simulink library "lib_fuel_cell"  (Simulink 4.00)
undefined symbols (not defined in the file or in its folder): air_cp, amb_tmp, cell_const_F, cell_const_g, cell_const_jo, cell_const_LHV_H2, cell_const_Mair, cell_const_MH, cell_const_MW, cell_const_R2, cell_const_Voc, ex_gas_cp, fan_cool, fc_acc_mass, fc_act, fc_air_comp_map, fc_air_comp_pwr, fc_base_mass, fc_blower_rec_H2, fc_blowera, fc_c2i_th_cond, fc_c_init_tmp, fc_cell_area, fc_cell_const_eta1, fc_cell_const_eta_DCDC, fc_cell_const_etablow, fc_cell_const_etagen, fc_cell_const_etapump, fc_cell_const_ex, fc_cell_const_kw, fc_cell_const_Nrad, fc_cell_const_U, fc_cell_dim_A, fc_cell_dim_tm, fc_cell_num, fc_cell_press_a, fc_cell_press_amb, fc_cell_press_an, fc_cell_press_blowa, fc_cell_press_blowr, fc_cell_press_c, fc_cell_press_hum, fc_cell_press_hyd, fc_cell_stack_dpipe, fc_cell_stack_dpipefc, fc_cell_stack_drad, fc_cell_stack_Lpipe, fc_cell_stack_Lpipefc, fc_cell_stack_Lrad, fc_cell_stack_N, fc_cell_stack_Pel, fc_cell_stoich_RHah, fc_cell_stoich_RHch, fc_cell_stoich_RHo, fc_cell_stoich_vH, fc_cell_stoich_vO, fc_cell_stoich_XON, fc_cell_temp_ah, fc_cell_temp_amb, fc_cell_temp_cell ... (+74)
libraries: fc_vt_lib x2, lib_fuel_cell x1
(part 2 of 5)

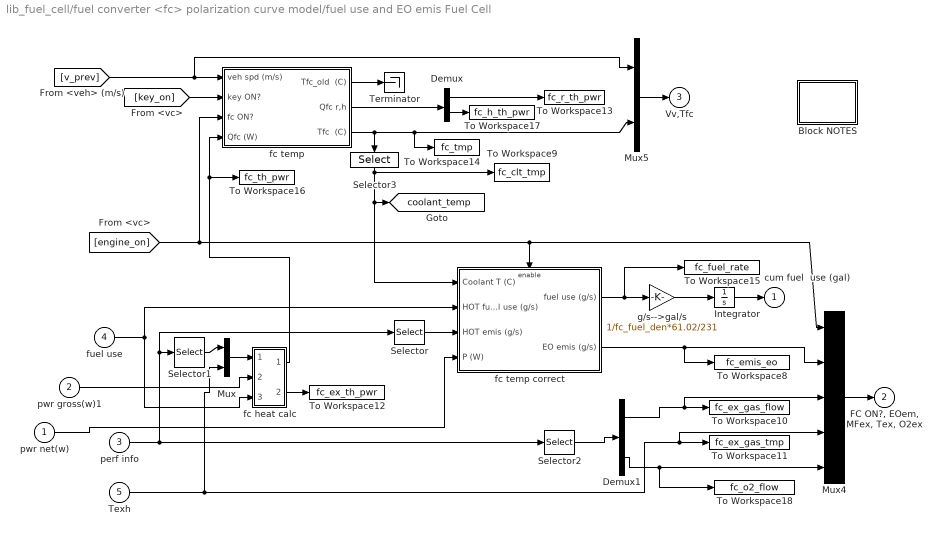
== system lib_fuel_cell/fuel converter <fc> polarization curve model/fuel use and EO emis Fuel Cell ==
  pwr net(w) : Inport  Port=1  LatchInput=off
  pwr gross(w)1 : Inport  Port=2  LatchInput=off
  perf info : Inport  Port=3  LatchInput=off
  fuel use : Inport  Port=4  LatchInput=off
  Texh : Inport  Port=5  LatchInput=off
  Block NOTES : Subsystem
      settings: RTWFcnNameOpts=Auto  RTWFileNameOpts=Auto
      mask Display: disp('Block\nNOTES')
  Demux : Demux  Outputs=2  BusSelectionMode=off
  Demux1 : Demux  Outputs=2  BusSelectionMode=off
  Integrator : Integrator  ExternalReset=none  InitialConditionSource=internal  InitialCondition=0  LimitOutput=off  UpperSaturationLimit=inf  LowerSaturationLimit=-inf  ShowSaturationPort=off  ShowStatePort=off  AbsoluteTolerance=auto
  Mux : Mux  Inputs=2
  Mux4 : Mux  Inputs=[1 4 1 1 1]
      settings: DisplayOption=none
  Mux5 : Mux  Inputs=[1 4 ]
      settings: DisplayOption=none
  Selector : Selector  InputType=Vector  ElementSrc=Internal  Elements=[1 2 3 4]  RowSrc=Internal  Rows=1  ColumnSrc=Internal  Columns=1  InputPortWidth=6
  Selector1 : Selector  InputType=Vector  ElementSrc=Internal  Elements=[5]  RowSrc=Internal  Rows=1  ColumnSrc=Internal  Columns=1  InputPortWidth=6
  Selector2 : Selector  InputType=Vector  ElementSrc=Internal  Elements=[5 6]  RowSrc=Internal  Rows=1  ColumnSrc=Internal  Columns=1  InputPortWidth=6
  Selector3 : Selector  Orientation=down  InputType=Vector  ElementSrc=Internal  Elements=2  RowSrc=Internal  Rows=1  ColumnSrc=Internal  Columns=1  InputPortWidth=4
  Terminator : Terminator
  To Workspace10 : ToWorkspace  VariableName=fc_ex_gas_flow  SampleTime=-1  SaveFormat=Array
  To Workspace11 : ToWorkspace  VariableName=fc_ex_gas_tmp  SampleTime=-1  SaveFormat=Array
  To Workspace12 : ToWorkspace  VariableName=fc_ex_th_pwr  SampleTime=-1  SaveFormat=Array
  To Workspace13 : ToWorkspace  VariableName=fc_r_th_pwr  SampleTime=-1  SaveFormat=Array
  To Workspace14 : ToWorkspace  VariableName=fc_tmp  SampleTime=-1  SaveFormat=Array
  To Workspace15 : ToWorkspace  VariableName=fc_fuel_rate  SampleTime=-1  SaveFormat=Array
  To Workspace16 : ToWorkspace  VariableName=fc_th_pwr  SampleTime=-1  SaveFormat=Array
  To Workspace17 : ToWorkspace  VariableName=fc_h_th_pwr  SampleTime=-1  SaveFormat=Array
  To Workspace18 : ToWorkspace  VariableName=fc_o2_flow  SampleTime=-1  SaveFormat=Array
  To Workspace8 : ToWorkspace  VariableName=fc_emis_eo  SampleTime=-1  SaveFormat=Array
  To Workspace9 : ToWorkspace  VariableName=fc_clt_tmp  SampleTime=-1  SaveFormat=Array
  fc heat calc : Subsystem
      settings: RTWFcnNameOpts=Auto  RTWFileNameOpts=Auto
  fc temp : Subsystem
      settings: RTWFcnNameOpts=Auto  RTWFileNameOpts=Auto
  fc temp correct : Subsystem  TreatAsAtomicUnit=on
      settings: RTWFcnNameOpts=Auto  RTWFileNameOpts=Auto
  g/s-->gal/s : Gain  Gain=1/fc_fuel_den*61.02/231  Multiplication=Element-wise(K.*u)  SaturateOnIntegerOverflow=on
  cum fuel  use (gal) : Outport  Port=1  InitialOutput=0
  "FC ON?, EOem, MFex, Tex, O2ex" : Outport  Port=2  InitialOutput=0
  Vv,Tfc : Outport  Port=3  InitialOutput=0
  tag scope: coolant_temp=global
  wires:
  perf info/1 -> Selector2/1, Selector/1, Selector1/1
  Selector/1 -> fc temp correct/3(HOT emis (g/s))
  fc temp correct/1(fuel use (g/s)) -> To Workspace15/1, g/s-->gal/s/1
  fc temp correct/2(EO emis (g/s)) -> To Workspace8/1, Mux4/2
  g/s-->gal/s/1 -> Integrator/1
  Selector3/1 -> To Workspace9/1, [coolant_temp], fc temp correct/1(Coolant T (C))
  [engine_on] -> fc temp/3(fc ON?), fc temp correct/Enable, Mux4/1
  Integrator/1 -> cum fuel  use (gal)/1
  Mux4/1 -> "FC ON?, EOem, MFex, Tex, O2ex"/1
  fuel use/1 -> fc temp correct/2(HOT fuel use (g/s)), fc heat calc/3(In4)
  [key_on] -> fc temp/2(key ON?)
  Demux/2 -> To Workspace17/1
  Demux/1 -> To Workspace13/1
  fc temp/2(Qfc r,h) -> Demux/1
  fc temp/1(Tfc_old  (C)) -> Terminator/1
  fc temp/3(Tfc  (C)) -> Mux5/2, To Workspace14/1, Selector3/1
  [v_prev] -> fc temp/1(veh spd (m/s)), Mux5/1
  Mux5/1 -> Vv,Tfc/1
  Selector2/1 -> Demux1/1
  Demux1/1 -> To Workspace10/1, Mux4/3
  Texh/1 -> To Workspace11/1, Mux4/4, Mux/2
  Demux1/2 -> To Workspace18/1, Mux4/5
  fc heat calc/2(Out1) -> To Workspace12/1
  fc heat calc/1(Out2) -> fc temp/4(Qfc (W)), To Workspace16/1
  Selector1/1 -> Mux/1
  Mux/1 -> fc heat calc/1(In5)
  pwr net(w)/1 -> fc temp correct/4(P (W))
  pwr gross(w)1/1 -> fc heat calc/2(In3)

== system lib_fuel_cell/fuel converter <fc>  KTH fc model/fuel cell  system <fc>/Block NOTES ==
  note: 7/30/98
      | - started with battery from BD_SER2h.m
      | - added a Saturation block to prevent computed
      |        SOC from falling below 0 or rising above 1
      | - added logic in 'limit power' to prevent discharge
      | if SOC is below 0.001 (0.1%)
      | -added limit block to check if low SOC is preventing
      | discharge
  note: Power loss is computed as I*R+losses due to Coulombic (in)efficiency.
  note: This block models the energy storage system as an SOC-dependent voltage
      | in series with an SOC- and current direction-dependent internal resistance.
      | SOC is computed assuming that A-h capacity is a function of average discharge
      | current:  (A-h capacity)=ess_peukert_coeff * (average discharge current)^ess_peukert_exp.
      |
      | Discharge power is limited here so as not to bring the bus (battery pack) voltage below
      | the minimum controller voltage and so as to allow the solution of the quadratic eq'n for
      | discharge current.
      |
      | Positive current is discharge current in the convention used here.

== system lib_fuel_cell/fuel converter <fc>  KTH fc model/fuel cell  system <fc>/KTH fc model ==
  note: KTH Fuel Cell System
      | (PEM Fuel Cell)
  note: W/ re-circulation of hydrogen
  In1 : Inport  Port=1  LatchInput=off
  Enable : EnablePort  StatesWhenEnabling=reset
  Fcn : Fcn  Expr=u(6)
  PEM fuel cell system : Subsystem
      settings: RTWFcnNameOpts=Auto  RTWFileNameOpts=Auto
  emissions info : Subsystem
      settings: RTWFcnNameOpts=Auto  RTWFileNameOpts=Auto
  pwr avail. to driveline (W) : Outport  Port=1  InitialOutput=0
  Emissions info : Outport  Port=2
  fuel use : Outport  Port=3  InitialOutput=0
  system characteristics : Outport  Port=4
  wires:
  In1/1 -> PEM fuel cell system/1("Power request from drivetrain [W] ")
  emissions info/1(emission info CO HC NOx PM mass flow exhaust exhaust temperature O2) -> Emissions info/1
  PEM fuel cell system/1(Pnet [W]) -> pwr avail. to driveline (W)/1
  PEM fuel cell system/2(System characteristics) -> Fcn/1, system characteristics/1
  Fcn/1 -> fuel use/1

== system lib_fuel_cell/fuel converter <fc>  KTH fc model/fuel use and EO emis Fuel Cell/Block NOTES ==
  note: This block determines actual fuel use and engine-out emissions
      | given the fully hot values and the engine coolant temperature.
      | The correlations used here were developed at NREL using
      | FTP data collected under subcontract by JDM & Associates.
      | Note: PM hot/cold relation assumed same as HC

== system lib_fuel_cell/fuel converter <fc> GCTool linkage/fuel cell  system <fc>/Block NOTES ==
  note: 7/30/98
      | - started with battery from BD_SER2h.m
      | - added a Saturation block to prevent computed
      |        SOC from falling below 0 or rising above 1
      | - added logic in 'limit power' to prevent discharge
      | if SOC is below 0.001 (0.1%)
      | -added limit block to check if low SOC is preventing
      | discharge
  note: Power loss is computed as I*R+losses due to Coulombic (in)efficiency.
  note: This block models the energy storage system as an SOC-dependent voltage
      | in series with an SOC- and current direction-dependent internal resistance.
      | SOC is computed assuming that A-h capacity is a function of average discharge
      | current:  (A-h capacity)=ess_peukert_coeff * (average discharge current)^ess_peukert_exp.
      |
      | Discharge power is limited here so as not to bring the bus (battery pack) voltage below
      | the minimum controller voltage and so as to allow the solution of the quadratic eq'n for
      | discharge current.
      |
      | Positive current is discharge current in the convention used here.

== system lib_fuel_cell/fuel converter <fc> GCTool linkage/fuel cell  system <fc>/GCTool fuel cell model ==
  note: Demux Port Labels:
      | net pwr (W)
      | hc (g/s)
      | co (g/s)
      | nox (g/s)
      | pm (g/s)
      | MFexh (g/s)
      | Texh (C)
      | O2 (g/s), dummy
      | ???
      | ???
      | ???
      | fuel use (kg/s)
  net pwr req (W) : Inport  Port=1  LatchInput=off
  Enable : EnablePort  StatesWhenEnabling=reset
  Demux : Demux  Outputs=11  BusSelectionMode=off
  GCTool  Fuel Cell Model : Subsystem  mask(GCTool Fuel Cell Model){x=1, y=2, z=3}
      mask prompts: x "param1:"; y "param2:"; z "param3:"
      mask help: This block will call the GCTool fuel cell modeling software to determine the output parameters of the fuel cell.
      settings: RTWFcnNameOpts=Auto  RTWFileNameOpts=Auto
  Ground : Ground
  Memory : Memory  Orientation=left  X0=[0 0 0]  InheritSampleTime=off
      settings: RTWStateStorageClass=Auto
  Mux5 : Mux  Inputs=7
      settings: DisplayOption=none
  Mux6 : Mux  Inputs=2
      settings: DisplayOption=none
  Mux7 : Mux  Inputs=3
      settings: DisplayOption=none
  net pwr out (W) : Outport  Port=1  OutputWhenDisabled=reset  InitialOutput=0
  emis info hc co nox pm MFexh Texh O2 : Outport  Port=2
  fuel use : Outport  Port=3  OutputWhenDisabled=reset  InitialOutput=0
  wires:
  Ground/1 -> Mux5/7
  Demux/11 -> fuel use/1
  Mux7/1 -> Memory/1
  Demux/10 -> Mux7/3
  Demux/9 -> Mux7/2
  Demux/8 -> Mux7/1
  Demux/7 -> Mux5/6
  Mux5/1 -> emis info hc co nox pm MFexh Texh O2/1
  Demux/6 -> Mux5/5
  Demux/5 -> Mux5/4
  Demux/4 -> Mux5/3
  Demux/3 -> Mux5/2
  Demux/2 -> Mux5/1
  Demux/1 -> net pwr out (W)/1
  Memory/1 -> Mux6/2
  Mux6/1 -> GCTool  Fuel Cell Model/1(In1)
  net pwr req (W)/1 -> Mux6/1
  GCTool  Fuel Cell Model/1(Out1) -> Demux/1

== system lib_fuel_cell/fuel converter <fc> GCTool linkage/fuel use and EO emis Fuel Cell/Block NOTES ==
  note: This block determines actual fuel use and engine-out emissions
      | given the fully hot values and the engine coolant temperature.
      | The correlations used here were developed at NREL using
      | FTP data collected under subcontract by JDM & Associates.
      | Note: PM hot/cold relation assumed same as HC

== system lib_fuel_cell/fuel converter <fc> GCTool linkage/fuel use and EO emis Fuel Cell/fc heat calc ==
  In5 : Inport  Port=1  LatchInput=off
  In3 : Inport  Port=2  LatchInput=off
  In4 : Inport  Port=3  LatchInput=off
  Fcn3 : Fcn  Expr=(u(1)/1000)*ex_gas_cp*(u(2) - amb_tmp)
  MinMax : MinMax  Function=min  Inputs=2
  Sum5 : Sum  Inputs=-+  SaturateOnIntegerOverflow=on
  Sum6 : Sum  Inputs=-+  SaturateOnIntegerOverflow=on
  lhv : Gain  Gain=fc_fuel_lhv  Multiplication=Element-wise(K.*u)  SaturateOnIntegerOverflow=on
  Out2 : Outport  Port=1  InitialOutput=0
  Out1 : Outport  Port=2  InitialOutput=0
  wires:
  In5/1 -> Fcn3/1
  Fcn3/1 -> MinMax/1
  Sum6/1 -> Sum5/2, MinMax/2
  lhv/1 -> Sum6/2
  Sum5/1 -> Out2/1
  In3/1 -> Sum6/1
  In4/1 -> lhv/1
  MinMax/1 -> Sum5/1, Out1/1

== system lib_fuel_cell/fuel converter <fc> GCTool linkage/fuel use and EO emis Fuel Cell/fc temp ==
  note: c
  note: i
  note: x
  note: h
  veh spd (m/s) : Inport  Port=1  LatchInput=off
  key ON? : Inport  Orientation=down  Port=2  LatchInput=off
  fc ON? : Inport  Port=3  LatchInput=off
  Qfc (W) : Inport  Port=4  LatchInput=off
  1/ : Gain  Gain=1/(0.2*fc_base_mass*fc_pwr_scale*fc_cp)  Multiplication=Element-wise(K.*u)  SaturateOnIntegerOverflow=on
  1/Ci : Gain  Gain=1/(0.8*fc_base_mass*fc_pwr_scale*fc_cp)  Multiplication=Element-wise(K.*u)  SaturateOnIntegerOverflow=on
  1/Cx : Gain  Gain=1/(fc_acc_mass*fc_pwr_scale*fc_cp)  Multiplication=Element-wise(K.*u)  SaturateOnIntegerOverflow=on
  1/mcp : Gain  Gain=1/(0.1*veh_glider_mass*fc_pwr_scale*fc_h_cp)  Multiplication=Element-wise(K.*u)  SaturateOnIntegerOverflow=on
  Block NOTES : Subsystem
      settings: RTWFcnNameOpts=Auto  RTWFileNameOpts=Auto
      mask Display: disp('Block\nNOTES')
  Mux3 : Mux  Inputs=4
      settings: DisplayOption=none
  Mux4 : Mux  Inputs=2
      settings: DisplayOption=none
  Qc : Sum  Inputs=++  SaturateOnIntegerOverflow=on
  Qc1 : Sum  Inputs=--+  SaturateOnIntegerOverflow=on
  Tcm : Integrator  ExternalReset=none  InitialConditionSource=internal  InitialCondition=fc_c_init_tmp  LimitOutput=off  UpperSaturationLimit=inf  LowerSaturationLimit=-inf  ShowSaturationPort=off  ShowStatePort=off  AbsoluteTolerance=auto
  Tcx : Integrator  ExternalReset=none  InitialConditionSource=internal  InitialCondition=fc_x_init_tmp  LimitOutput=off  UpperSaturationLimit=inf  LowerSaturationLimit=-inf  ShowSaturationPort=off  ShowStatePort=off  AbsoluteTolerance=auto
  Tcx1 : Integrator  ExternalReset=none  InitialConditionSource=internal  InitialCondition=fc_i_init_tmp  LimitOutput=off  UpperSaturationLimit=inf  LowerSaturationLimit=-inf  ShowSaturationPort=off  ShowStatePort=off  AbsoluteTolerance=auto
  Tm : Integrator  ExternalReset=none  InitialConditionSource=internal  InitialCondition=fc_h_init_tmp  LimitOutput=off  UpperSaturationLimit=inf  LowerSaturationLimit=-inf  ShowSaturationPort=off  ShowStatePort=off  AbsoluteTolerance=auto
  fc coolant : Subsystem  TreatAsAtomicUnit=on
      settings: RTWFcnNameOpts=Auto  RTWFileNameOpts=Auto
  fc mass heat flow : Subsystem
      settings: RTWFcnNameOpts=Auto  RTWFileNameOpts=Auto
  old fc coolant  temp. (C) : Subsystem
      settings: RTWFcnNameOpts=Auto  RTWFileNameOpts=Auto
  Tfc_old  (C) : Outport  Port=1  InitialOutput=0
  Qfc r,h : Outport  Port=2  InitialOutput=0
  Tfc  (C) : Outport  Port=3  InitialOutput=0
  wires:
  fc ON?/1 -> old fc coolant  temp. (C)/1(fc on?)
  veh spd (m/s)/1 -> fc mass heat flow/1(veh spd), old fc coolant  temp. (C)/2(veh spd)
  old fc coolant  temp. (C)/1(fc coolant  temp (C)) -> Tfc_old  (C)/1
  Mux3/1 -> Tfc  (C)/1, fc mass heat flow/2(fc_temp)
  fc mass heat flow/4(Qfc_h) -> 1/mcp/1
  1/mcp/1 -> Tm/1
  Tm/1 -> Mux3/4
  Tcx/1 -> Mux3/3
  key ON?/1 -> fc coolant/Enable
  fc mass heat flow/3(Qfc_x) -> 1/Cx/1
  1/Cx/1 -> Tcx/1
  Mux4/1 -> Qfc r,h/1
  Tcx1/1 -> Mux3/2, fc coolant/1(Tcl)
  fc coolant/1(Qfc_rad) -> Mux4/1, Qc1/1
  fc coolant/2(Qfc_htr) -> Mux4/2, Qc1/2
  fc mass heat flow/2(Qfc_i) -> fc coolant/2("Qfc_i "), Qc1/3
  Tcm/1 -> Mux3/1
  1/Ci/1 -> Tcx1/1
  Qc1/1 -> 1/Ci/1
  fc mass heat flow/1(Qfc_c) -> Qc/2
  Qfc (W)/1 -> Qc/1
  1//1 -> Tcm/1
  Qc/1 -> 1//1

== system lib_fuel_cell/fuel converter <fc> VT model/Fuel Cell Power System Model (S. Gurski - Virgina Tech)/Algebraic Constraint1 ==
  f(z) : Inport  Port=1  LatchInput=off
  Initial Guess : InitialCondition  Value=z0
  Sum : Sum  Inputs=|++  SaturateOnIntegerOverflow=on
  z : Outport  Port=1
  wires:
  Sum/1 -> Initial Guess/1
  Initial Guess/1 -> Sum/2, z/1
  f(z)/1 -> Sum/1

== system lib_fuel_cell/fuel converter <fc> VT model/Fuel Cell Power System Model (S. Gurski - Virgina Tech)/Bus Creator ==
  In1 : Inport  Port=1  LatchInput=off
  Bus Creator : BusCreator  Inputs=59
  Demux : Demux  Outputs=59  BusSelectionMode=off
  system_characteristics : Outport  Port=1
  wires:
  Demux/30 -> Bus Creator/30  "water_balance"
  Demux/29 -> Bus Creator/29  "condenser_working_capacity"
  Demux/28 -> Bus Creator/28  "cell_voltage"
  Demux/23 -> Bus Creator/23  "mwv_anode_inlet"
  Demux/24 -> Bus Creator/24  "mwv_cathode_inlet"
  Demux/25 -> Bus Creator/25  "water_gen"
  Demux/26 -> Bus Creator/26  "mwv_cathode_outlet"
  Demux/27 -> Bus Creator/27  "condenser_recovered_water"
  Demux/1 -> Bus Creator/1  "fc_gross_power_gen"
  Demux/2 -> Bus Creator/2  "air_compressor_power"
  Demux/3 -> Bus Creator/3  "condenser_fan_power"
  Demux/4 -> Bus Creator/4  "radiator_fan_power"
  Demux/5 -> Bus Creator/5  "coolant_pump_power"
  Demux/6 -> Bus Creator/6  "m_dot_air"
  Demux/7 -> Bus Creator/7  "m_dot_coolant"
  Demux/8 -> Bus Creator/8  "pressure_inlet_cathode"
  Demux/9 -> Bus Creator/9  "fc_cell_current"
  Demux/10 -> Bus Creator/10  "m_dot_h2"
  Demux/11 -> Bus Creator/11  "q_gen_stack"
  Demux/12 -> Bus Creator/12  "t_stack_coolant_in"
  Demux/13 -> Bus Creator/13  "t_stack_coolant_output"
  Demux/14 -> Bus Creator/14  "t_humidifier_coolant_out"
  Demux/15 -> Bus Creator/15  "t_radiator_coolant_out"
  Demux/16 -> Bus Creator/16  "condenser_heat_to_ambient"
  Demux/17 -> Bus Creator/17  "radiator_energy_loss_ambient"
  Demux/18 -> Bus Creator/18  "stack_energy_loss_ambient"
  Demux/19 -> Bus Creator/19  "reservoir_energy_loss_ambient"
  Demux/20 -> Bus Creator/20  "air_compressor_speed"
  Demux/21 -> Bus Creator/21  "air_compressor_adiabatic_efficiency"
  Demux/22 -> Bus Creator/22  "air_compressor_volumetric_efficiency"
  In1/1 -> Demux/1
  Bus Creator/1 -> system_characteristics/1
  Demux/31 -> Bus Creator/31  "condensed_water_in_stack"
  Demux/32 -> Bus Creator/32  "m_dot_h2o_anode"
  Demux/33 -> Bus Creator/33  "m_dot_h2o_cathode"
  Demux/34 -> Bus Creator/34  "stack_heat_loads1"
  Demux/35 -> Bus Creator/35  "stack_heat_loads2"
  Demux/36 -> Bus Creator/36  "stack_heat_loads3"
  Demux/37 -> Bus Creator/37  "stack_heat_loads4"
  Demux/38 -> Bus Creator/38  "stack_heat_loads5"
  Demux/39 -> Bus Creator/39  "stack_heat_loads6"
  Demux/40 -> Bus Creator/40  "stack_heat_loads7"
  Demux/41 -> Bus Creator/41  "stack_heat_loads8"
  Demux/42 -> Bus Creator/42  "stack_heat_loads9"
  Demux/43 -> Bus Creator/43  "Q_humidifier"
  Demux/44 -> Bus Creator/44  "cell_efficiency"
  Demux/45 -> Bus Creator/45  "system_efficiency"
  Demux/46 -> Bus Creator/46  "exhaust_m_dot_water"
  Demux/47 -> Bus Creator/47  "exhaust_heat_loss"
  Demux/48 -> Bus Creator/48  "exhaust_quality"
  Demux/49 -> Bus Creator/49  "oxygen_partial_pressure"
  Demux/50 -> Bus Creator/50  "pressure_ratio"
  Demux/51 -> Bus Creator/51  "operating_pressure"
  Demux/52 -> Bus Creator/52  "m_dot_air_out"
  Demux/53 -> Bus Creator/53  "by_pass_energy_loss_ambient"
  Demux/54 -> Bus Creator/54  "o2_pp_inlet"
  Demux/55 -> Bus Creator/55  "o2_pp_outlet"
  Demux/56 -> Bus Creator/56  "psat"
  Demux/57 -> Bus Creator/57  "t_compresser_out"
  Demux/58 -> Bus Creator/58  "t_reservoir_coolant_out"
  Demux/59 -> Bus Creator/59  "o2_percent"

== system lib_fuel_cell/fuel converter <fc> VT model/Fuel Cell Power System Model (S. Gurski - Virgina Tech)/Fuel Cell System ==
  In1 : Inport  Port=1  LatchInput=off
  Action Port : ActionPort  InitializeStates=held  ActionType=unset
  Algebraic Constraint : Subsystem  AncestorBlock=simulink3/Math/Algebraic Constraint  mask(Algebraic Constraint){z0=0.3}
      mask prompts: z0 "Initial guess:"
      mask help: Constrains input signal f(z) to zero and outputs an algebraic state z. This block outputs the value necessary to produce a zero at the input. The output must affect the input through some feedback path. Provide an initial guess of the output to improve algebraic loop solver efficiency.
      settings: RTWFcnNameOpts=Auto  RTWFileNameOpts=Auto
      mask Help:
      | This block outputs the value necessary to produce a zero at the input. The output must affect the input through some feedback path. This allows you to specify algebraic equations for index 1 differential/algebraic systems (DAE's).
      | 
      | By default, the initial guess is zero.  You can improve the efficiency of the algebraic loop solver by providing an initial guess that is close to the solution value.
      mask Display: disp('Solve\nf(z) = 0')
  Constant : Constant  Value=1
  Demux1 : Demux  Outputs=6  BusSelectionMode=off
  Fuel Cell System : Subsystem
      settings: RTWFcnNameOpts=Auto  RTWFileNameOpts=Auto
  Mux : Mux  Inputs=6
  Sum : Sum  Inputs=|+-  SaturateOnIntegerOverflow=on
  Out1 : Outport  Port=1  OutputWhenDisabled=reset  InitialOutput=0
  Out2 : Outport  Port=2  OutputWhenDisabled=reset  InitialOutput=0
  wires:
  Algebraic Constraint/1(z) -> Fuel Cell System/1(" Current Density Request")
  Sum/1 -> Algebraic Constraint/1(f(z))
  Mux/1 -> Out1/1
  In1/1 -> Demux1/1
  Demux1/1 -> Sum/1
  Demux1/2 -> Fuel Cell System/2(t_stack_coolant_in1)
  Demux1/3 -> Fuel Cell System/3(fc_stack_temperature)
  Demux1/4 -> Fuel Cell System/4(water_balance_previous)
  Fuel Cell System/1(Net Power Gen) -> Mux/1, Sum/2
  Fuel Cell System/2(Stack Temperature) -> Mux/2
  Fuel Cell System/3(cell_voltage) -> Mux/3
  Fuel Cell System/4(t_stack_coolant_in) -> Mux/4
  Fuel Cell System/5(waterbalance) -> Mux/5
  Constant/1 -> Out2/1
  Fuel Cell System/6(system_characteristics) -> Mux/6
  Demux1/5 -> Fuel Cell System/5(elevation)
  Demux1/6 -> Fuel Cell System/6(vehicle speed (m/s))

== system lib_fuel_cell/fuel converter <fc> VT model/Fuel Cell Power System Model (S. Gurski - Virgina Tech)/Fuel Cell System - min voltage ==
  " Current Density Request" : Inport  Port=1  LatchInput=off
  t_stack_coolant_in1 : Inport  Port=2  LatchInput=off
  fc_stack_temperature : Inport  Port=3  LatchInput=off
  water_balance_previous : Inport  Port=4  LatchInput=off
  elevation : Inport  Port=5  LatchInput=off
  vehicle speed (m/s) : Inport  Port=6  LatchInput=off
  Main Loop - min voltage : fc_vt_lib/Main Loop - min voltage
      settings: RTWFcnNameOpts=Auto  RTWFileNameOpts=Auto
  Net Power Gen : Outport  Port=1
  Stack Temperature : Outport  Port=2
  cell_voltage : Outport  Port=3
  t_stack_coolant_in : Outport  Port=4
  waterbalance : Outport  Port=5
  system_characteristics : Outport  Port=6
  wires:
  elevation/1 -> Main Loop - min voltage/5
  Main Loop - min voltage/6 -> system_characteristics/1
  water_balance_previous/1 -> Main Loop - min voltage/4
  fc_stack_temperature/1 -> Main Loop - min voltage/3
  t_stack_coolant_in1/1 -> Main Loop - min voltage/2
  Main Loop - min voltage/5 -> cell_voltage/1
  " Current Density Request"/1 -> Main Loop - min voltage/1
  Main Loop - min voltage/2 -> waterbalance/1
  Main Loop - min voltage/3 -> Stack Temperature/1
  Main Loop - min voltage/4 -> t_stack_coolant_in/1
  Main Loop - min voltage/1 -> Net Power Gen/1
  vehicle speed (m/s)/1 -> Main Loop - min voltage/6

== system lib_fuel_cell/fuel converter <fc> VT model/fuel use and EO emis Fuel Cell/Block NOTES ==
  note: This block determines actual fuel use and engine-out emissions
      | given the fully hot values and the engine coolant temperature.
      | The correlations used here were developed at NREL using
      | FTP data collected under subcontract by JDM & Associates.
      | Note: PM hot/cold relation assumed same as HC

== system lib_fuel_cell/fuel converter <fc> net model/fuel cell  system <fc>/Block NOTES ==
  note: 7/30/98
      | - started with battery from BD_SER2h.m
      | - added a Saturation block to prevent computed
      |        SOC from falling below 0 or rising above 1
      | - added logic in 'limit power' to prevent discharge
      | if SOC is below 0.001 (0.1%)
      | -added limit block to check if low SOC is preventing
      | discharge
  note: Power loss is computed as I*R+losses due to Coulombic (in)efficiency.
  note: This block models the energy storage system as an SOC-dependent voltage
      | in series with an SOC- and current direction-dependent internal resistance.
      | SOC is computed assuming that A-h capacity is a function of average discharge
      | current:  (A-h capacity)=ess_peukert_coeff * (average discharge current)^ess_peukert_exp.
      |
      | Discharge power is limited here so as not to bring the bus (battery pack) voltage below
      | the minimum controller voltage and so as to allow the solution of the quadratic eq'n for
      | discharge current.
      |
      | Positive current is discharge current in the convention used here.

== system lib_fuel_cell/fuel converter <fc> net model/fuel cell  system <fc>/pwr vs. eff  fuel cell model ==
  net pwr req (W) : Inport  Port=1  LatchInput=off
  Enable : EnablePort  StatesWhenEnabling=reset
  enforce limits : Subsystem
      settings: RTWFcnNameOpts=Auto  RTWFileNameOpts=Auto
  net pwr avail (W) : Outport  Port=1  OutputWhenDisabled=reset  InitialOutput=0
  wires:
  enforce limits/1(Out1) -> net pwr avail (W)/1
  net pwr req (W)/1 -> enforce limits/1(In1)

== system lib_fuel_cell/fuel converter <fc> net model/fuel use and EO emis Fuel Cell/Block NOTES ==
  note: This block determines actual fuel use and engine-out emissions
      | given the fully hot values and the engine coolant temperature.
      | The correlations used here were developed at NREL using
      | FTP data collected under subcontract by JDM & Associates.
      | Note: PM hot/cold relation assumed same as HC

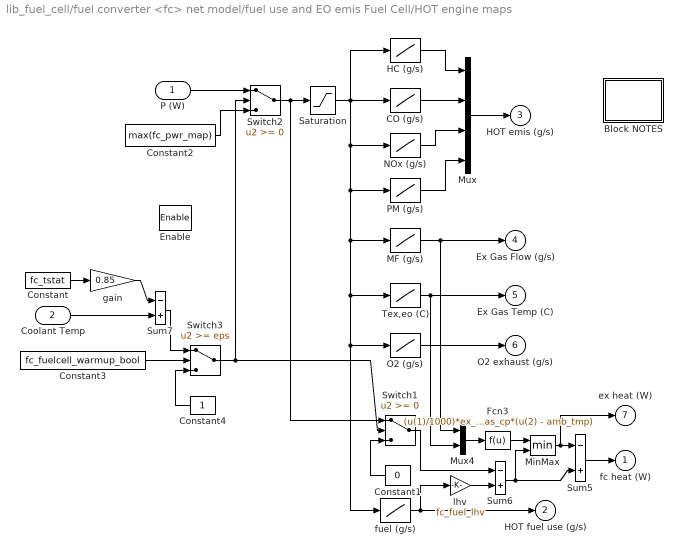
== system lib_fuel_cell/fuel converter <fc> net model/fuel use and EO emis Fuel Cell/HOT engine maps  ==
  P (W) : Inport  Port=1  LatchInput=off
  Coolant Temp : Inport  Port=2  LatchInput=off
  Enable : EnablePort  StatesWhenEnabling=reset
  Block NOTES : Subsystem
      settings: RTWFcnNameOpts=Auto  RTWFileNameOpts=Auto
      mask Display: disp('Block\nNOTES')
  CO (g/s) : Lookup  InputValues=fc_pwr_map*fc_pwr_scale  OutputValues=fc_co_map*fc_pwr_scale
  Constant : Constant  Value=fc_tstat
  Constant1 : Constant  Orientation=left  Value=0
  Constant2 : Constant  Value=max(fc_pwr_map)
  Constant3 : Constant  Value=fc_fuelcell_warmup_bool
  Constant4 : Constant  Orientation=left  Value=1
  Fcn3 : Fcn  Expr=(u(1)/1000)*ex_gas_cp*(u(2) - amb_tmp)
  HC (g/s) : Lookup  InputValues=fc_pwr_map*fc_pwr_scale  OutputValues=fc_hc_map*fc_pwr_scale
  MF (g/s) : Lookup  InputValues=fc_pwr_map*fc_pwr_scale  OutputValues=fc_exflow_map*fc_pwr_scale
  MinMax : MinMax  Function=min  Inputs=2
  Mux : Mux  Inputs=4
      settings: DisplayOption=none
  Mux4 : Mux  Inputs=2
      settings: DisplayOption=none
  NOx (g/s) : Lookup  InputValues=fc_pwr_map*fc_pwr_scale  OutputValues=fc_nox_map*fc_pwr_scale
  O2 (g/s) : Lookup  InputValues=fc_pwr_map*fc_pwr_scale  OutputValues=fc_o2_map*fc_pwr_scale
  PM (g/s) : Lookup  InputValues=fc_pwr_map*fc_pwr_scale  OutputValues=fc_pm_map*fc_pwr_scale
  Saturation : Saturate  UpperLimit=max(fc_pwr_map*fc_pwr_scale)  LowerLimit=0  LinearizeAsGain=on
  Sum5 : Sum  Inputs=-+  SaturateOnIntegerOverflow=on
  Sum6 : Sum  Inputs=-+  SaturateOnIntegerOverflow=on
  Sum7 : Sum  Inputs=-+  SaturateOnIntegerOverflow=on
  Switch1 : Switch  Threshold=0
  Switch2 : Switch  Threshold=0
  Switch3 : Switch  Threshold=eps
  Tex,eo (C) : Lookup  InputValues=fc_pwr_map*fc_pwr_scale  OutputValues=fc_extmp_map
  fuel (g/s) : Lookup  InputValues=fc_pwr_map*fc_pwr_scale  OutputValues=fc_fuel_map*fc_pwr_scale/fc_eff_scale
  gain : Gain  Gain=0.85  Multiplication=Element-wise(K.*u)  SaturateOnIntegerOverflow=on
  lhv : Gain  Gain=fc_fuel_lhv  Multiplication=Element-wise(K.*u)  SaturateOnIntegerOverflow=on
  fc heat (W) : Outport  Port=1  OutputWhenDisabled=reset  InitialOutput=eps
  HOT fuel use (g/s) : Outport  Port=2  OutputWhenDisabled=reset  InitialOutput=eps
  HOT emis (g/s) : Outport  Port=3  OutputWhenDisabled=reset  InitialOutput=eps
  Ex Gas Flow (g/s) : Outport  Port=4  OutputWhenDisabled=reset  InitialOutput=eps
  Ex Gas Temp (C) : Outport  Port=5  OutputWhenDisabled=reset  InitialOutput=amb_tmp
  O2 exhaust (g/s) : Outport  Port=6  OutputWhenDisabled=reset  InitialOutput=eps
  ex heat (W) : Outport  Port=7  OutputWhenDisabled=reset  InitialOutput=eps
  wires:
  O2 (g/s)/1 -> O2 exhaust (g/s)/1
  fuel (g/s)/1 -> lhv/1, HOT fuel use (g/s)/1
  Constant1/1 -> Switch1/3
  lhv/1 -> Sum6/2
  Sum6/1 -> MinMax/2, Sum5/2
  MinMax/1 -> ex heat (W)/1, Sum5/1
  Fcn3/1 -> MinMax/1
  Sum5/1 -> fc heat (W)/1
  Mux4/1 -> Fcn3/1
  Switch1/1 -> Sum6/1
  CO (g/s)/1 -> Mux/2
  Saturation/1 -> HC (g/s)/1, NOx (g/s)/1, PM (g/s)/1, O2 (g/s)/1, fuel (g/s)/1, Tex,eo (C)/1, MF (g/s)/1, CO (g/s)/1
  Tex,eo (C)/1 -> Mux4/2, Ex Gas Temp (C)/1
  MF (g/s)/1 -> Mux4/1, Ex Gas Flow (g/s)/1
  Mux/1 -> HOT emis (g/s)/1
  NOx (g/s)/1 -> Mux/3
  HC (g/s)/1 -> Mux/1
  PM (g/s)/1 -> Mux/4
  P (W)/1 -> Switch2/1
  Constant2/1 -> Switch2/3
  Switch2/1 -> Saturation/1, Switch1/1
  Switch3/1 -> Switch1/2, Switch2/2
  Constant3/1 -> Switch3/2
  Sum7/1 -> Switch3/1
  gain/1 -> Sum7/1
  Coolant Temp/1 -> Sum7/2
  Constant/1 -> gain/1
  Constant4/1 -> Switch3/3

== system lib_fuel_cell/fuel converter <fc> net model/fuel use and EO emis Fuel Cell/System  Efficiency ==
  In1 : Inport  Port=1  LatchInput=off
  Constant : Constant  Value=eps
  Gain : Gain  Gain=fc_fuel_lhv  Multiplication=Element-wise(K.*u)  SaturateOnIntegerOverflow=on
  Gain1 : Gain  Gain=100  Multiplication=Element-wise(K.*u)  SaturateOnIntegerOverflow=on
  Product : Product  Inputs=*/  Multiplication=Element-wise(.*)  SaturateOnIntegerOverflow=on
  Sum1 : Sum  Inputs=|++  SaturateOnIntegerOverflow=on
  To Workspace1 : ToWorkspace  VariableName=fc_eff_out_a  SampleTime=-1  SaveFormat=Array
  tag scope: fc_eff_out_a=global
  wires:
  [fc_pwr_out_a] -> Product/1
  Product/1 -> Gain1/1
  Gain/1 -> Sum1/1
  Constant/1 -> Sum1/2
  Sum1/1 -> Product/2
  Gain1/1 -> To Workspace1/1, [fc_eff_out_a]
  In1/1 -> Gain/1

== system lib_fuel_cell/fuel converter <fc> net model/fuel use and EO emis Fuel Cell/fc temp ==
  note: c
  note: i
  note: x
  note: h
  veh spd (m/s) : Inport  Port=1  LatchInput=off
  key ON? : Inport  Orientation=down  Port=2  LatchInput=off
  fc ON? : Inport  Port=3  LatchInput=off
  Qfc (W) : Inport  Port=4  LatchInput=off
  1/ : Gain  Gain=1/(0.2*fc_base_mass*fc_pwr_scale*fc_cp)  Multiplication=Element-wise(K.*u)  SaturateOnIntegerOverflow=on
  1/Ci : Gain  Gain=1/(0.8*fc_base_mass*fc_pwr_scale*fc_cp)  Multiplication=Element-wise(K.*u)  SaturateOnIntegerOverflow=on
  1/Cx : Gain  Gain=1/(fc_acc_mass*fc_pwr_scale*fc_cp)  Multiplication=Element-wise(K.*u)  SaturateOnIntegerOverflow=on
  1/mcp : Gain  Gain=1/(0.1*veh_glider_mass*fc_pwr_scale*fc_h_cp)  Multiplication=Element-wise(K.*u)  SaturateOnIntegerOverflow=on
  Block NOTES : Subsystem
      settings: RTWFcnNameOpts=Auto  RTWFileNameOpts=Auto
      mask Display: disp('Block\nNOTES')
  Mux3 : Mux  Inputs=4
      settings: DisplayOption=none
  Mux4 : Mux  Inputs=2
      settings: DisplayOption=none
  Qc : Sum  Inputs=++  SaturateOnIntegerOverflow=on
  Qc1 : Sum  Inputs=--+  SaturateOnIntegerOverflow=on
  Tcm : Integrator  ExternalReset=none  InitialConditionSource=internal  InitialCondition=fc_c_init_tmp  LimitOutput=off  UpperSaturationLimit=inf  LowerSaturationLimit=-inf  ShowSaturationPort=off  ShowStatePort=off  AbsoluteTolerance=auto
  Tcx : Integrator  ExternalReset=none  InitialConditionSource=internal  InitialCondition=fc_x_init_tmp  LimitOutput=off  UpperSaturationLimit=inf  LowerSaturationLimit=-inf  ShowSaturationPort=off  ShowStatePort=off  AbsoluteTolerance=auto
  Tcx1 : Integrator  ExternalReset=none  InitialConditionSource=internal  InitialCondition=fc_i_init_tmp  LimitOutput=off  UpperSaturationLimit=inf  LowerSaturationLimit=-inf  ShowSaturationPort=off  ShowStatePort=off  AbsoluteTolerance=auto
  Tm : Integrator  ExternalReset=none  InitialConditionSource=internal  InitialCondition=fc_h_init_tmp  LimitOutput=off  UpperSaturationLimit=inf  LowerSaturationLimit=-inf  ShowSaturationPort=off  ShowStatePort=off  AbsoluteTolerance=auto
  fc coolant : Subsystem  TreatAsAtomicUnit=on
      settings: RTWFcnNameOpts=Auto  RTWFileNameOpts=Auto
  fc mass heat flow : Subsystem
      settings: RTWFcnNameOpts=Auto  RTWFileNameOpts=Auto
  old fc coolant  temp. (C) : Subsystem
      settings: RTWFcnNameOpts=Auto  RTWFileNameOpts=Auto
  Tfc_old  (C) : Outport  Port=1  InitialOutput=0
  Qfc r,h : Outport  Port=2  InitialOutput=0
  Tfc  (C) : Outport  Port=3  InitialOutput=0
  wires:
  fc ON?/1 -> old fc coolant  temp. (C)/1(fc on?)
  veh spd (m/s)/1 -> fc mass heat flow/1(veh spd), old fc coolant  temp. (C)/2(veh spd)
  old fc coolant  temp. (C)/1(fc coolant  temp (C)) -> Tfc_old  (C)/1
  Mux3/1 -> Tfc  (C)/1, fc mass heat flow/2(fc_temp)
  fc mass heat flow/4(Qfc_h) -> 1/mcp/1
  1/mcp/1 -> Tm/1
  Tm/1 -> Mux3/4
  Tcx/1 -> Mux3/3
  key ON?/1 -> fc coolant/Enable
  fc mass heat flow/3(Qfc_x) -> 1/Cx/1
  1/Cx/1 -> Tcx/1
  Mux4/1 -> Qfc r,h/1
  Tcx1/1 -> Mux3/2, fc coolant/1(Tcl)
  fc coolant/1(Qfc_rad) -> Mux4/1, Qc1/1
  fc coolant/2(Qfc_htr) -> Mux4/2, Qc1/2
  fc mass heat flow/2(Qfc_i) -> fc coolant/2("Qfc_i "), Qc1/3
  Tcm/1 -> Mux3/1
  1/Ci/1 -> Tcx1/1
  Qc1/1 -> 1/Ci/1
  fc mass heat flow/1(Qfc_c) -> Qc/2
  Qfc (W)/1 -> Qc/1
  1//1 -> Tcm/1
  Qc/1 -> 1//1

== system lib_fuel_cell/fuel converter <fc> net model/fuel use and EO emis Fuel Cell/fc temp correct ==
  Coolant T (C) : Inport  Port=1  LatchInput=off
  HOT fuel use (g/s) : Inport  Port=2  LatchInput=off
  HOT emis (g/s) : Inport  Port=3  LatchInput=off
  P (W) : Inport  Port=4  LatchInput=off
  Enable : EnablePort  StatesWhenEnabling=reset
  =1: use map based =0: use constant equation based : Constant  Value=fc_cold
  Switch : Switch  Threshold=eps
  Switch1 : Switch  Threshold=eps
  fc temp correct Constant Correction Factors (Equation Based) : Subsystem  TreatAsAtomicUnit=on
      settings: RTWFcnNameOpts=Auto  RTWFileNameOpts=Auto
  fc temp correct Variable Correction Factors (Map Based) : Subsystem  TreatAsAtomicUnit=on
      settings: RTWFcnNameOpts=Auto  RTWFileNameOpts=Auto
  fc_cold=0 : Logic  Operator=NOT  Inputs=2
  fuel use (g/s) : Outport  Port=1  OutputWhenDisabled=reset  InitialOutput=0
  EO emis (g/s) : Outport  Port=2  OutputWhenDisabled=reset  InitialOutput=0
  wires:
  P (W)/1 -> fc temp correct Variable Correction Factors (Map Based)/4(P (W))
  =1: use map based =0: use constant equation based/1 -> fc_cold=0/1, fc temp correct Variable Correction Factors (Map Based)/Enable
  Coolant T (C)/1 -> fc temp correct Constant Correction Factors (Equation Based)/1(Coolant T (C)), fc temp correct Variable Correction Factors (Map Based)/1(Coolant T (C))
  HOT fuel use (g/s)/1 -> fc temp correct Constant Correction Factors (Equation Based)/2(HOT fuel use (g/s)), fc temp correct Variable Correction Factors (Map Based)/2(HOT fuel use (g/s))
  HOT emis (g/s)/1 -> fc temp correct Constant Correction Factors (Equation Based)/3(HOT emis (g/s)), fc temp correct Variable Correction Factors (Map Based)/3(HOT emis (g/s))
  fc temp correct Constant Correction Factors (Equation Based)/1(fuel use (g/s)) -> Switch/1
  fc_cold=0/1 -> fc temp correct Constant Correction Factors (Equation Based)/Enable, Switch/2, Switch1/2
  fc temp correct Variable Correction Factors (Map Based)/1(fuel use (g/s)) -> Switch/3
  fc temp correct Constant Correction Factors (Equation Based)/2(EO emis (g/s)) -> Switch1/1
  fc temp correct Variable Correction Factors (Map Based)/2(EO emis (g/s)) -> Switch1/3
  Switch/1 -> fuel use (g/s)/1
  Switch1/1 -> EO emis (g/s)/1

== system lib_fuel_cell/fuel converter <fc> polarization curve model/fuel cell  system <fc>/Block NOTES ==
  note: 7/30/98
      | - started with battery from BD_SER2h.m
      | - added a Saturation block to prevent computed
      |        SOC from falling below 0 or rising above 1
      | - added logic in 'limit power' to prevent discharge
      | if SOC is below 0.001 (0.1%)
      | -added limit block to check if low SOC is preventing
      | discharge
  note: Power loss is computed as I*R+losses due to Coulombic (in)efficiency.
  note: This block models the energy storage system as an SOC-dependent voltage
      | in series with an SOC- and current direction-dependent internal resistance.
      | SOC is computed assuming that A-h capacity is a function of average discharge
      | current:  (A-h capacity)=ess_peukert_coeff * (average discharge current)^ess_peukert_exp.
      |
      | Discharge power is limited here so as not to bring the bus (battery pack) voltage below
      | the minimum controller voltage and so as to allow the solution of the quadratic eq'n for
      | discharge current.
      |
      | Positive current is discharge current in the convention used here.

== system lib_fuel_cell/fuel converter <fc> polarization curve model/fuel cell  system <fc>/Diagnostics ==
  In1 : Inport  Port=1  LatchInput=off
  In2 : Inport  Port=2  LatchInput=off
  Demux1 : Demux  Outputs=11  BusSelectionMode=off
  Fuel usage (g/s)1 : ToWorkspace  VariableName=fc_fuel_pump_pwr_out_a  SampleTime=-1  SaveFormat=Array
  Fuel usage (g/s)2 : ToWorkspace  VariableName=fc_air_comp_pwr_out_a  SampleTime=-1  SaveFormat=Array
  Fuel usage (g/s)3 : ToWorkspace  VariableName=fc_coolant_pump_pwr_out_a  SampleTime=-1  SaveFormat=Array
  Fuel usage (g/s)4 : ToWorkspace  VariableName=fc_water_pump_pwr_out_a  SampleTime=-1  SaveFormat=Array
  To Workspace1 : ToWorkspace  VariableName=fc_gross_pwr_out_a  SampleTime=-1  SaveFormat=Array
  To Workspace10 : ToWorkspace  VariableName=fc_cell_I_out_a  SampleTime=-1  SaveFormat=Array
  To Workspace11 : ToWorkspace  VariableName=fc_cell_V_out_a  SampleTime=-1  SaveFormat=Array
  To Workspace12 : ToWorkspace  VariableName=fc_V_out_a  SampleTime=-1  SaveFormat=Array
  To Workspace13 : ToWorkspace  VariableName=fc_I_out_a  SampleTime=-1  SaveFormat=Array
  To Workspace14 : ToWorkspace  VariableName=fc_gross_pwr_out_r  SampleTime=-1  SaveFormat=Array
  To Workspace15 : ToWorkspace  VariableName=fc_excess_fuel_a  SampleTime=-1  SaveFormat=Array
  To Workspace16 : ToWorkspace  VariableName=fc_cell_crrnt_den_out_a  SampleTime=-1  SaveFormat=Array
  wires:
  Demux1/2 -> To Workspace16/1
  Demux1/3 -> To Workspace10/1
  Demux1/4 -> To Workspace13/1
  Demux1/5 -> To Workspace11/1
  Demux1/6 -> To Workspace12/1
  In1/1 -> Demux1/1
  Demux1/7 -> To Workspace15/1
  Demux1/1 -> To Workspace14/1
  In2/1 -> To Workspace1/1
  Demux1/8 -> Fuel usage (g/s)1/1
  Demux1/9 -> Fuel usage (g/s)2/1
  Demux1/10 -> Fuel usage (g/s)4/1
  Demux1/11 -> Fuel usage (g/s)3/1

== system lib_fuel_cell/fuel converter <fc> polarization curve model/fuel cell  system <fc>/polarization curve fuel cell model ==
  pwr req  (W) : Inport  Port=1  LatchInput=off
  Enable : EnablePort  StatesWhenEnabling=reset
  Auxilaries  (actual) : Subsystem
      settings: RTWFcnNameOpts=Auto  RTWFileNameOpts=Auto
  Auxilaries  (estimated) : Subsystem
      settings: RTWFcnNameOpts=Auto  RTWFileNameOpts=Auto
  Fuel Cell Stack : Subsystem
      settings: RTWFcnNameOpts=Auto  RTWFileNameOpts=Auto
  Mux : Mux  Inputs=[7 4]
  Selector1 : Selector  InputType=Vector  ElementSrc=Internal  Elements=[6]  RowSrc=Internal  Rows=1  ColumnSrc=Internal  Columns=1  InputPortWidth=7
  Selector2 : Selector  InputType=Vector  ElementSrc=Internal  Elements=[1 2 3 4 5 7]  RowSrc=Internal  Rows=1  ColumnSrc=Internal  Columns=1  InputPortWidth=7
  Sum : Sum  Inputs=+-  SaturateOnIntegerOverflow=on
  prev fuel (g/s) : Memory  Orientation=left  X0=(cyc_mph(1,2)>0)*mean(fc_fuel_map)*fc_pwr_scale/fc_eff_scale  InheritSampleTime=off
      settings: RTWStateStorageClass=Auto
  pwr sum1 : Sum  Inputs=2  SaturateOnIntegerOverflow=on
  pwr out a (W) Net : Outport  Port=1  OutputWhenDisabled=reset  InitialOutput=0
  pwr out a (W) Gross1 : Outport  Port=2  OutputWhenDisabled=reset  InitialOutput=0
  emis info hc co nox pm MFexh O2 : Outport  Port=3  OutputWhenDisabled=reset  InitialOutput=[0 0 0 0 0 0]
  fuel use g/s : Outport  Port=4  OutputWhenDisabled=reset  InitialOutput=0
  "emis info Texh " : Outport  Port=5  InitialOutput=amb_tmp
  diagnostics : Outport  Port=6  OutputWhenDisabled=reset  InitialOutput=[0 0 0 0 0 0 0 0 0 0 0]
  wires:
  Fuel Cell Stack/2(fuel used (g/s)) -> fuel use g/s/1, prev fuel (g/s)/1, Auxilaries  (actual)/1(In1)
  pwr req  (W)/1 -> pwr sum1/1
  Auxilaries  (actual)/1(Out1) -> Sum/2
  pwr sum1/1 -> Fuel Cell Stack/1(Pack pwr req)
  prev fuel (g/s)/1 -> Auxilaries  (estimated)/1(prev fuel  req (g/s))
  Auxilaries  (estimated)/1(Aux pwr req'd (W)) -> pwr sum1/2
  Fuel Cell Stack/3(emis info) -> Selector2/1, Selector1/1
  Selector2/1 -> emis info hc co nox pm MFexh O2/1
  Selector1/1 -> "emis info Texh "/1
  Sum/1 -> pwr out a (W) Net/1
  Fuel Cell Stack/1(gross pwr out a (W)) -> Sum/1, pwr out a (W) Gross1/1
  Mux/1 -> diagnostics/1
  Fuel Cell Stack/4(diagnostics) -> Mux/1
  Auxilaries  (actual)/2(Out2) -> Mux/2

== system lib_fuel_cell/fuel converter <fc> polarization curve model/fuel use and EO emis Fuel Cell/Block NOTES ==
  note: This block determines actual fuel use and engine-out emissions
      | given the fully hot values and the engine coolant temperature.
      | The correlations used here were developed at NREL using
      | FTP data collected under subcontract by JDM & Associates.
      | Note: PM hot/cold relation assumed same as HC

== system lib_fuel_cell/fuel converter <fc> polarization curve model/fuel use and EO emis Fuel Cell/fc heat calc ==
  In5 : Inport  Port=1  LatchInput=off
  In3 : Inport  Port=2  LatchInput=off
  In4 : Inport  Port=3  LatchInput=off
  Fcn3 : Fcn  Expr=(u(1)/1000)*ex_gas_cp*(u(2) - amb_tmp)
  MinMax : MinMax  Function=min  Inputs=2
  Sum5 : Sum  Inputs=-+  SaturateOnIntegerOverflow=on
  Sum6 : Sum  Inputs=-+  SaturateOnIntegerOverflow=on
  lhv : Gain  Gain=fc_fuel_lhv  Multiplication=Element-wise(K.*u)  SaturateOnIntegerOverflow=on
  Out2 : Outport  Port=1  InitialOutput=0
  Out1 : Outport  Port=2  InitialOutput=0
  wires:
  In5/1 -> Fcn3/1
  Fcn3/1 -> MinMax/1
  Sum6/1 -> Sum5/2, MinMax/2
  lhv/1 -> Sum6/2
  Sum5/1 -> Out2/1
  In3/1 -> Sum6/1
  In4/1 -> lhv/1
  MinMax/1 -> Sum5/1, Out1/1

== system lib_fuel_cell/fuel converter <fc> polarization curve model/fuel use and EO emis Fuel Cell/fc temp ==
  note: c
  note: i
  note: x
  note: h
  veh spd (m/s) : Inport  Port=1  LatchInput=off
  key ON? : Inport  Orientation=down  Port=2  LatchInput=off
  fc ON? : Inport  Port=3  LatchInput=off
  Qfc (W) : Inport  Port=4  LatchInput=off
  1/ : Gain  Gain=1/(0.2*fc_base_mass*fc_pwr_scale*fc_cp)  Multiplication=Element-wise(K.*u)  SaturateOnIntegerOverflow=on
  1/Ci : Gain  Gain=1/(0.8*fc_base_mass*fc_pwr_scale*fc_cp)  Multiplication=Element-wise(K.*u)  SaturateOnIntegerOverflow=on
  1/Cx : Gain  Gain=1/(fc_acc_mass*fc_pwr_scale*fc_cp)  Multiplication=Element-wise(K.*u)  SaturateOnIntegerOverflow=on
  1/mcp : Gain  Gain=1/(0.1*veh_glider_mass*fc_pwr_scale*fc_h_cp)  Multiplication=Element-wise(K.*u)  SaturateOnIntegerOverflow=on
  Block NOTES : Subsystem
      settings: RTWFcnNameOpts=Auto  RTWFileNameOpts=Auto
      mask Display: disp('Block\nNOTES')
  Mux3 : Mux  Inputs=4
      settings: DisplayOption=none
  Mux4 : Mux  Inputs=2
      settings: DisplayOption=none
  Qc : Sum  Inputs=++  SaturateOnIntegerOverflow=on
  Qc1 : Sum  Inputs=--+  SaturateOnIntegerOverflow=on
  Tcm : Integrator  ExternalReset=none  InitialConditionSource=internal  InitialCondition=fc_c_init_tmp  LimitOutput=off  UpperSaturationLimit=inf  LowerSaturationLimit=-inf  ShowSaturationPort=off  ShowStatePort=off  AbsoluteTolerance=auto
  Tcx : Integrator  ExternalReset=none  InitialConditionSource=internal  InitialCondition=fc_x_init_tmp  LimitOutput=off  UpperSaturationLimit=inf  LowerSaturationLimit=-inf  ShowSaturationPort=off  ShowStatePort=off  AbsoluteTolerance=auto
  Tcx1 : Integrator  ExternalReset=none  InitialConditionSource=internal  InitialCondition=fc_i_init_tmp  LimitOutput=off  UpperSaturationLimit=inf  LowerSaturationLimit=-inf  ShowSaturationPort=off  ShowStatePort=off  AbsoluteTolerance=auto
  Tm : Integrator  ExternalReset=none  InitialConditionSource=internal  InitialCondition=fc_h_init_tmp  LimitOutput=off  UpperSaturationLimit=inf  LowerSaturationLimit=-inf  ShowSaturationPort=off  ShowStatePort=off  AbsoluteTolerance=auto
  fc coolant : Subsystem  TreatAsAtomicUnit=on
      settings: RTWFcnNameOpts=Auto  RTWFileNameOpts=Auto
  fc mass heat flow : Subsystem
      settings: RTWFcnNameOpts=Auto  RTWFileNameOpts=Auto
  old fc coolant  temp. (C) : Subsystem
      settings: RTWFcnNameOpts=Auto  RTWFileNameOpts=Auto
  Tfc_old  (C) : Outport  Port=1  InitialOutput=0
  Qfc r,h : Outport  Port=2  InitialOutput=0
  Tfc  (C) : Outport  Port=3  InitialOutput=0
  wires:
  fc ON?/1 -> old fc coolant  temp. (C)/1(fc on?)
  veh spd (m/s)/1 -> fc mass heat flow/1(veh spd), old fc coolant  temp. (C)/2(veh spd)
  old fc coolant  temp. (C)/1(fc coolant  temp (C)) -> Tfc_old  (C)/1
  Mux3/1 -> Tfc  (C)/1, fc mass heat flow/2(fc_temp)
  fc mass heat flow/4(Qfc_h) -> 1/mcp/1
  1/mcp/1 -> Tm/1
  Tm/1 -> Mux3/4
  Tcx/1 -> Mux3/3
  key ON?/1 -> fc coolant/Enable
  fc mass heat flow/3(Qfc_x) -> 1/Cx/1
  1/Cx/1 -> Tcx/1
  Mux4/1 -> Qfc r,h/1
  Tcx1/1 -> Mux3/2, fc coolant/1(Tcl)
  fc coolant/1(Qfc_rad) -> Mux4/1, Qc1/1
  fc coolant/2(Qfc_htr) -> Mux4/2, Qc1/2
  fc mass heat flow/2(Qfc_i) -> fc coolant/2("Qfc_i "), Qc1/3
  Tcm/1 -> Mux3/1
  1/Ci/1 -> Tcx1/1
  Qc1/1 -> 1/Ci/1
  fc mass heat flow/1(Qfc_c) -> Qc/2
  Qfc (W)/1 -> Qc/1
  1//1 -> Tcm/1
  Qc/1 -> 1//1

== system lib_fuel_cell/fuel converter <fc> polarization curve model/fuel use and EO emis Fuel Cell/fc temp correct ==
  Coolant T (C) : Inport  Port=1  LatchInput=off
  HOT fuel use (g/s) : Inport  Port=2  LatchInput=off
  HOT emis (g/s) : Inport  Port=3  LatchInput=off
  P (W) : Inport  Port=4  LatchInput=off
  Enable : EnablePort  StatesWhenEnabling=reset
  =1: use map based =0: use constant equation based : Constant  Value=fc_cold
  Switch : Switch  Threshold=eps
  Switch1 : Switch  Threshold=eps
  fc temp correct Constant Correction Factors (Equation Based) : Subsystem  TreatAsAtomicUnit=on
      settings: RTWFcnNameOpts=Auto  RTWFileNameOpts=Auto
  fc temp correct Variable Correction Factors (Map Based) : Subsystem  TreatAsAtomicUnit=on
      settings: RTWFcnNameOpts=Auto  RTWFileNameOpts=Auto
  fc_cold=0 : Logic  Operator=NOT  Inputs=2
  fuel use (g/s) : Outport  Port=1  OutputWhenDisabled=reset  InitialOutput=0
  EO emis (g/s) : Outport  Port=2  OutputWhenDisabled=reset  InitialOutput=0
  wires:
  P (W)/1 -> fc temp correct Variable Correction Factors (Map Based)/4(P (W))
  =1: use map based =0: use constant equation based/1 -> fc_cold=0/1, fc temp correct Variable Correction Factors (Map Based)/Enable
  Coolant T (C)/1 -> fc temp correct Constant Correction Factors (Equation Based)/1(Coolant T (C)), fc temp correct Variable Correction Factors (Map Based)/1(Coolant T (C))
  HOT fuel use (g/s)/1 -> fc temp correct Constant Correction Factors (Equation Based)/2(HOT fuel use (g/s)), fc temp correct Variable Correction Factors (Map Based)/2(HOT fuel use (g/s))
  HOT emis (g/s)/1 -> fc temp correct Constant Correction Factors (Equation Based)/3(HOT emis (g/s)), fc temp correct Variable Correction Factors (Map Based)/3(HOT emis (g/s))
  fc temp correct Constant Correction Factors (Equation Based)/1(fuel use (g/s)) -> Switch/1
  fc_cold=0/1 -> fc temp correct Constant Correction Factors (Equation Based)/Enable, Switch/2, Switch1/2
  fc temp correct Variable Correction Factors (Map Based)/1(fuel use (g/s)) -> Switch/3
  fc temp correct Constant Correction Factors (Equation Based)/2(EO emis (g/s)) -> Switch1/1
  fc temp correct Variable Correction Factors (Map Based)/2(EO emis (g/s)) -> Switch1/3
  Switch/1 -> fuel use (g/s)/1
  Switch1/1 -> EO emis (g/s)/1
